simulink model "VCU_board_v8"  (R2019b)
settings: Solver=VariableStepAuto  StartTime=0.0  StopTime=300  RelTol=1e-3
undefined symbols (not defined in the file): canChannel
libraries: canmsglib x46, canlib x40
(part 2 of 2)

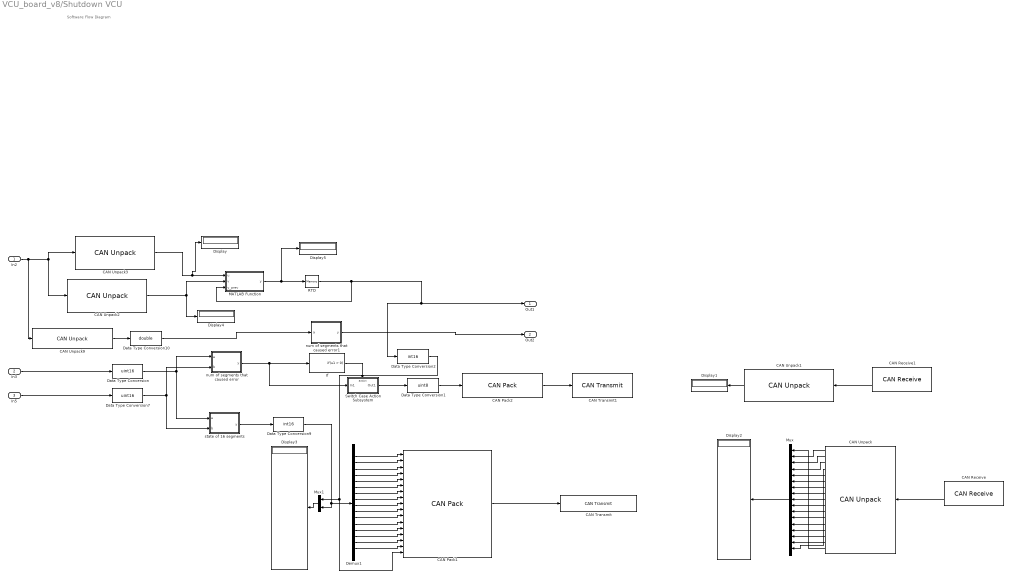
== system VCU_board_v8/Shutdown VCU ==
  note: Software Flow Diagram
  In2 : Inport
  In3 : Inport  Port=2
  In5 : Inport  Port=3
  CAN Pack1 : canmsglib/CAN Pack  MsgList=(none)  MsgName=CAN Msg  MsgIDType=Standard (11-bit identifier)  MsgIdentifier=22  MsgLength=3  Remote=off  ApplyMinMax=off  BusOutput=off  SignalInfo={ 'Signal1/DashLED1', '8', '1', 'LE', 'unsigned', 'Standard', '0', '1', '0', '-Inf', 'Inf'; 'Signal2/DashLED2', '9', '1', 'LE', 'unsigned', 'Standard', '0', '1', '0', '-Inf', 'Inf'; 'Signal3/DashLED3', '10', '1', 'LE', 'unsigned', 'Standard', '0', '1', '0', '-Inf', 'Inf'; 'Signal4/DashLED4', '11', '1', 'LE', 'unsigned', 'Standard', '0', '1', '0', '-Inf', 'Inf'; 'Signal5', '12', '1', 'LE', 'unsigned', 'Standard', '0', '1', '0', '-Inf', 'Inf'; 'Signal6', '13', '1', 'LE', 'unsigned', 'Standard', '0', '1', '0', '-Inf', 'Inf'; 'Signal7', '14', '1', 'LE', 'unsigned', 'Standard', '0', '1', '0', '-Inf', 'Inf'; 'Signal8', '15', '1', 'LE', 'unsigned', 'Standard', '0', '1', '0', '-Inf', 'Inf'; 'Signal9', '16', '1', 'LE', 'unsigned', 'Standard', '0', '1', '0', '-Inf', 'Inf'; 'Signal10', '17', '1', 'LE', 'unsigned', 'Standard', '0', '1', '0', '-Inf', 'Inf'; 'Signal11', '18', '1', 'LE', 'unsigned', 'Standard', '0', '1', '0', '-Inf', 'Inf'; 'Signal12', '19', '1', 'LE', 'unsigned', 'Standard', '0', '1', '0', '-Inf', 'Inf'; 'Signal13', '20', '1', 'LE', 'unsigned', 'Standard', '0', '1', '0', '-Inf', 'Inf'; 'Signal14', '21', '1', 'LE', 'unsigned', 'Standard', '0', '1', '0', '-Inf', 'Inf'; 'Signal15', '22', '1', 'LE', 'unsigned', 'Standard', '0', '1', '0', '-Inf', 'Inf'; 'Signal16', '23', '1', 'LE', 'unsigned', 'Standard', '0', '1', '0', '-Inf', 'Inf'; 'Accumulator FAN', '0', '1', 'LE', 'unsigned', 'Standard', '0', '1', '0', '-Inf', 'Inf' }
      settings: SourceProductName=Vehicle Network Toolbox  SourceProductBaseCode=VN  DataFormat=manually specified signals
  CAN Pack2 : canmsglib/CAN Pack  MsgList=(none)  MsgName=CAN Msg  MsgIDType=Standard (11-bit identifier)  MsgIdentifier=21  MsgLength=1  Remote=off  ApplyMinMax=off  BusOutput=off  SignalInfo={ 'Signal1', '0', '3', 'LE', 'unsigned', 'Standard', '0', '1', '0', '-Inf', 'Inf' }
      settings: SourceProductName=Vehicle Network Toolbox  SourceProductBaseCode=VN  DataFormat=manually specified signals
  CAN Receive : canlib/CAN Receive  BlockHandle=386.0002  Device=MathWorks Virtual 1 (Channel 1)  DeviceMenu=MathWorks Virtual 1 (Channel 1)  ObjConstructor=canChannel('MathWorks', 'Virtual 1', 1)  EnableStandardIDsFilter=off  StdIDsCombo=Allow all  StandardIDs=1  EnableExtendedIDsFilter=off  ExtIDsCombo=Allow all  ExtendedIDs=0  SampleTime=0.01  MsgsPerTimestep=all  InternalFilterUpdateStatus=on  BusOutput=off
      settings: SourceProductName=Vehicle Network Toolbox  SourceProductBaseCode=VN
  CAN Receive1 : canlib/CAN Receive  BlockHandle=387.0002  Device=MathWorks Virtual 1 (Channel 1)  DeviceMenu=MathWorks Virtual 1 (Channel 1)  ObjConstructor=canChannel('MathWorks', 'Virtual 1', 1)  EnableStandardIDsFilter=off  StdIDsCombo=Allow all  StandardIDs=1  EnableExtendedIDsFilter=off  ExtIDsCombo=Allow all  ExtendedIDs=0  SampleTime=0.01  MsgsPerTimestep=all  InternalFilterUpdateStatus=on  BusOutput=off
      settings: SourceProductName=Vehicle Network Toolbox  SourceProductBaseCode=VN
  CAN Transmit : canlib/CAN Transmit  BlockHandle=388.0002  Device=MathWorks Virtual 1 (Channel 1)  DeviceMenu=MathWorks Virtual 1 (Channel 1)  ObjConstructor=canChannel('MathWorks', 'Virtual 1', 1)  EnablePeriodicTransmit=on  MessagePeriod=0.250
      settings: SourceProductName=Vehicle Network Toolbox  SourceProductBaseCode=VN
  CAN Transmit1 : canlib/CAN Transmit  BlockHandle=389.0002  Device=MathWorks Virtual 1 (Channel 1)  DeviceMenu=MathWorks Virtual 1 (Channel 1)  ObjConstructor=canChannel('MathWorks', 'Virtual 1', 1)  EnablePeriodicTransmit=on  MessagePeriod=0.250
      settings: SourceProductName=Vehicle Network Toolbox  SourceProductBaseCode=VN
  CAN Unpack : canmsglib/CAN Unpack  MsgList=(none)  MsgName=CAN Msg  MsgIDType=Standard (11-bit identifier)  MsgIdentifier=22  MsgLength=3  SignalInfo={ 'Signal1', '8', '1', 'LE', 'unsigned', 'Standard', '0', '1', '0', '-Inf', 'Inf'; 'Signal2', '9', '1', 'LE', 'unsigned', 'Standard', '0', '1', '0', '-Inf', 'Inf'; 'Signal3', '10', '1', 'LE', 'unsigned', 'Standard', '0', '1', '0', '-Inf', 'Inf'; 'Signal4', '11', '1', 'LE', 'unsigned', 'Standard', '0', '1', '0', '-Inf', 'Inf'; 'Signal5', '12', '1', 'LE', 'unsigned', 'Standard', '0', '1', '0', '-Inf', 'Inf'; 'Signal6', '13', '1', 'LE', 'unsigned', 'Standard', '0', '1', '0', '-Inf', 'Inf'; 'Signal7', '14', '1', 'LE', 'unsigned', 'Standard', '0', '1', '0', '-Inf', 'Inf'; 'Signal8', '15', '1', 'LE', 'unsigned', 'Standard', '0', '1', '0', '-Inf', 'Inf'; 'Signal9', '16', '1', 'LE', 'unsigned', 'Standard', '0', '1', '0', '-Inf', 'Inf'; 'Signal10', '17', '1', 'LE', 'unsigned', 'Standard', '0', '1', '0', '-Inf', 'Inf'; 'Signal11', '18', '1', 'LE', 'unsigned', 'Standard', '0', '1', '0', '-Inf', 'Inf'; 'Signal12', '19', '1', 'LE', 'unsigned', 'Standard', '0', '1', '0', '-Inf', 'Inf'; 'Signal13', '20', '1', 'LE', 'unsigned', 'Standard', '0', '1', '0', '-Inf', 'Inf'; 'Signal14', '21', '1', 'LE', 'unsigned', 'Standard', '0', '1', '0', '-Inf', 'Inf'; 'Signal15', '22', '1', 'LE', 'unsigned', 'Standard', '0', '1', '0', '-Inf', 'Inf'; 'Signal16', '23', '1', 'LE', 'unsigned', 'Standard', '0', '1', '0', '-Inf', 'Inf'; 'Accumulator FAN', '0', '1', 'LE', 'unsigned', 'Standard', '0', '1', '0', '-Inf', 'Inf' }  IDPort=off  TimestampPort=off  ErrorPort=off  RemotePort=off  LengthPort=off  StatusPort=off  ApplyMinMax=off
      settings: SourceProductName=Vehicle Network Toolbox  SourceProductBaseCode=VN
  CAN Unpack1 : canmsglib/CAN Unpack  MsgList=(none)  MsgName=CAN Msg  MsgIDType=Standard (11-bit identifier)  MsgIdentifier=21  MsgLength=1  SignalInfo={ 'Signal1', '0', '3', 'LE', 'unsigned', 'Standard', '0', '1', '0', '-Inf', 'Inf' }  IDPort=off  TimestampPort=off  ErrorPort=off  RemotePort=off  LengthPort=off  StatusPort=off  ApplyMinMax=off
      settings: SourceProductName=Vehicle Network Toolbox  SourceProductBaseCode=VN
  CAN Unpack2 : canmsglib/CAN Unpack  MsgList=(none)  MsgName=Reset Notif  MsgIDType=Standard (11-bit identifier)  MsgIdentifier=61  MsgLength=1  SignalInfo={ 'Reset', '0', '1', 'LE', 'unsigned', 'Standard', '0', '1', '0', '-Inf', 'Inf' }  IDPort=off  TimestampPort=off  ErrorPort=off  RemotePort=off  LengthPort=off  StatusPort=off  ApplyMinMax=off
      settings: SourceProductName=Vehicle Network Toolbox  SourceProductBaseCode=VN
  CAN Unpack3 : canmsglib/CAN Unpack  MsgList=(none)  MsgName=Reset Notif  MsgIDType=Standard (11-bit identifier)  MsgIdentifier=41  MsgLength=3  SignalInfo={ 'Reset', '0', '1', 'LE', 'unsigned', 'Standard', '0', '1', '0', '-Inf', 'Inf' }  IDPort=off  TimestampPort=off  ErrorPort=off  RemotePort=off  LengthPort=off  StatusPort=off  ApplyMinMax=off
      settings: SourceProductName=Vehicle Network Toolbox  SourceProductBaseCode=VN
  CAN Unpack9 : canmsglib/CAN Unpack  MsgList=(none)  MsgName=CAN Msg  MsgIDType=Standard (11-bit identifier)  MsgIdentifier=51  MsgLength=6  SignalInfo={ 'Signal1', '24', '12', 'LE', 'unsigned', 'Standard', '0', '1', '0', '-Inf', 'Inf' }  IDPort=off  TimestampPort=off  ErrorPort=off  RemotePort=off  LengthPort=off  StatusPort=off  ApplyMinMax=off
      settings: SourceProductName=Vehicle Network Toolbox  SourceProductBaseCode=VN
  Data Type Conversion : DataTypeConversion  OutDataTypeStr=uint16
  Data Type Conversion1 : DataTypeConversion  OutDataTypeStr=uint8
  Data Type Conversion10 : DataTypeConversion  OutDataTypeStr=double
  Data Type Conversion2 : DataTypeConversion  OutDataTypeStr=int16
  Data Type Conversion7 : DataTypeConversion  OutDataTypeStr=uint16
  Data Type Conversion9 : DataTypeConversion  OutDataTypeStr=int16
  Demux1 : Demux  Outputs=16
  Display{,1..5} (6 alike) : Display
  If : If  ShowElse=off
  MATLAB Function : MATLAB Function  TreatAsAtomicUnit=on
  Mux : Mux  Inputs=17
  Mux1 : Mux  Inputs=2
  RTD : Memory  InheritSampleTime=on
  Switch Case Action Subsystem : Subsystem  TreatAsAtomicUnit=on
  num of segments that caused error : MATLAB Function  TreatAsAtomicUnit=on
  num of segments that caused error1 : MATLAB Function  TreatAsAtomicUnit=on
  state of 16 segments : MATLAB Function  TreatAsAtomicUnit=on
  Out1 : Outport
  Out2 : Outport  Port=2
  wires:
  CAN Pack1/1 -> CAN Transmit/1
  Data Type Conversion7/1 -> state of 16 segments/2(b), num of segments that caused error/2(b)
  Demux1/9 -> CAN Pack1/9
  Demux1/2 -> CAN Pack1/2
  CAN Unpack/9 -> Mux/10
  CAN Unpack/2 -> Mux/3
  CAN Unpack/4 -> Mux/5
  CAN Unpack/3 -> Mux/4
  Demux1/11 -> CAN Pack1/11
  CAN Unpack/6 -> Mux/7
  Demux1/3 -> CAN Pack1/3
  Demux1/5 -> CAN Pack1/5
  Demux1/16 -> CAN Pack1/16
  Demux1/15 -> CAN Pack1/15
  Demux1/12 -> CAN Pack1/12
  CAN Unpack9/1 -> Data Type Conversion10/1
  If/1 -> Switch Case Action Subsystem/Action
  Demux1/13 -> CAN Pack1/13
  Data Type Conversion9/1 -> Mux1/2, Demux1/1
  num of segments that caused error/1(y) -> If/1, Switch Case Action Subsystem/1(In1)
  Demux1/7 -> CAN Pack1/7
  state of 16 segments/1(y) -> Data Type Conversion9/1
  CAN Pack2/1 -> CAN Transmit1/1
  Data Type Conversion2/1 -> CAN Pack1/17, Mux1/1
  Demux1/8 -> CAN Pack1/8
  num of segments that caused error1/1(y) -> Out2/1
  Data Type Conversion1/1 -> CAN Pack2/1
  Mux1/1 -> Display3/1
  CAN Unpack/13 -> Mux/14
  CAN Unpack/8 -> Mux/9
  Mux/1 -> Display2/1
  Demux1/10 -> CAN Pack1/10
  CAN Receive1/2 -> CAN Unpack1/1
  Demux1/6 -> CAN Pack1/6
  CAN Unpack/7 -> Mux/8
  CAN Unpack/5 -> Mux/6
  In3/1 -> Data Type Conversion/1
  Data Type Conversion10/1 -> num of segments that caused error1/1(a)
  Switch Case Action Subsystem/1(Out1) -> Data Type Conversion1/1
  Demux1/14 -> CAN Pack1/14
  Demux1/4 -> CAN Pack1/4
  CAN Unpack/15 -> Mux/16
  CAN Unpack/16 -> Mux/17
  CAN Unpack/14 -> Mux/15
  CAN Unpack/12 -> Mux/13
  CAN Unpack/11 -> Mux/12
  Demux1/1 -> CAN Pack1/1
  CAN Unpack/17 -> Mux/1
  CAN Receive/2 -> CAN Unpack/1
  In5/1 -> Data Type Conversion7/1
  CAN Unpack/1 -> Mux/2
  CAN Unpack/10 -> Mux/11
  Data Type Conversion/1 -> num of segments that caused error/1(a), state of 16 segments/1(a)
  CAN Unpack1/1 -> Display1/1
  In2/1 -> CAN Unpack9/1, CAN Unpack3/1, CAN Unpack2/1
  CAN Unpack2/1 -> Display4/1, MATLAB Function/2(v)
  MATLAB Function/1(y) -> Display5/1, RTD/1
  RTD/1 -> MATLAB Function/3(y_prev), Out1/1, Data Type Conversion2/1
  CAN Unpack3/1 -> Display/1, MATLAB Function/1(u)

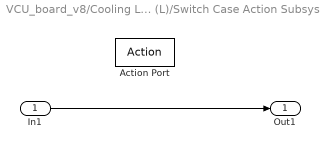
== system VCU_board_v8/Cooling Loop VCU (L)/Switch Case Action Subsystem ==
  In1 : Inport
  Action Port : ActionPort  ActionPortLabel=if(u1 > 150)
  Out1 : Outport
  wires:
  In1/1 -> Out1/1

== system VCU_board_v8/Cooling Loop VCU (R)/Switch Case Action Subsystem ==
  In1 : Inport
  Action Port : ActionPort  ActionPortLabel=if(u1 > 150)
  Out1 : Outport
  wires:
  In1/1 -> Out1/1

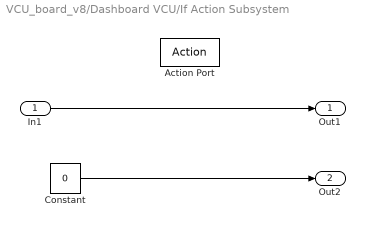
== system VCU_board_v8/Dashboard VCU/If Action Subsystem ==
  In1 : Inport
  Action Port : ActionPort  ActionPortLabel=if(u1 == 1)
  Constant : Constant  Value=0  OutDataTypeStr=boolean
  Out1 : Outport
  Out2 : Outport  Port=2
  wires:
  In1/1 -> Out1/1
  Constant/1 -> Out2/1

== system VCU_board_v8/Shutdown VCU/Switch Case Action Subsystem ==
  In1 : Inport
  Action Port : ActionPort  ActionPortLabel=if(u1 > 0)
  Out1 : Outport
  wires:
  In1/1 -> Out1/1

== matlab function VCU_board_v8/Shutdown VCU/state of 16 segments ==
  data: a input; y output; b input
function y = fcn(a,b)
c = [1,1,1,1,1,1,1,1,1,1,1,1,1,1,1,1];


for i=1:length(a)
   if a(i) ~= b(i)
        c(i) = 0;
   end
end
y = c;
end

== matlab function VCU_board_v8/Shutdown VCU/num of segments that caused error ==
  data: a input; y output; b input
function y = fcn(a,b)
c = [1,1,1,1,1,1,1,1,1,1,1,1,1,1,1,1];
count = 0;

for i=1:length(a)
   if a(i) ~= b(i)
        c(i) = 0;
        count = count + 1;
   end
end
y = count;
end

== matlab function VCU_board_v8/Brakebox VCU/Compare Accel Values ==
  data: u input; y output; v input
function y = accelcompare(u, v)
% Checks if there is 12% difference or greater and returns 1 if true

if (v <  u*1.1 ) && (v > u*0.9 )
    y = 0;  
    return
end
y = 1;



end

== matlab function VCU_board_v8/Dashboard VCU/Loop to work out logic ==
  data: RTD input; RTD2 output; Btn input; Reset input; Brake input; Siren output; LED output; Reset2 output
function [RTD2,Siren,LED,Reset2] = DashboardLogic(RTD, Btn, Reset, Brake)

if (RTD == 1)
    if (Btn == 1)
        RTD2 = 1;
        Siren = 1;
        LED = 1;
        Reset2 = 0;
    else % Btn == 0
        RTD2 = 1;
        Siren = 0;
        LED = 1;
        Reset2 = 0;
    end
else % RTD == 0
    if (Reset == 1)
        if (Brake == 1)
            if (Btn == 1)
                RTD2 = 1;
                Siren = 0;
                LED = 1; % In this scenario LED would flash
                Reset2 = 0;
            else % Btn == 0
                RTD2 = 0;
                Siren = 0;
                LED = 1;
                Reset2 = 1;
            end
        else % Brake == 0
            RTD2 = 0;
            Siren = 0;
            LED = 0;
            Reset2 = 1;
        end
    else % Reset == 0
        RTD2 = 0;
        Siren = 0;
        LED = 0;
        Reset2 = 0;
    end
end



end

== matlab function VCU_board_v8/Shutdown VCU/num of segments that caused error1 ==
  data: a input; y output
function y = fcn(a)
    if a > 0
        y= 1;
        return
    end
    y= 0;

end

== matlab function VCU_board_v8/Shutdown VCU/MATLAB Function ==
  data: u input; y output; v input; y_prev input
function y = fcn(u, v, y_prev)

if (u == 1)
    y = 1;
elseif (v == 1)
    y = 0;
else
    y = y_prev;
end

== matlab function VCU_board_v8/Cooling Loop VCU (R)/MATLAB Function ==
  data: u input; y output; v input; y_prev input
function y = fcn(u, v, y_prev)

if (u == 1)
    y = 1;
elseif (v == 1)
    y = 0;
else
    y = y_prev;
end

== matlab function VCU_board_v8/Cooling Loop VCU (L)/MATLAB Function ==
  data: u input; y output; v input; y_prev input
function y = fcn(u, v, y_prev)

if (u == 1)
    y = 1;
elseif (v == 1)
    y = 0;
else
    y = y_prev;
end
